simulink model "series"  (R2020a)
settings: Solver=VariableStepAuto  StartTime=0.0  StopTime=5  RelTol=1e-3
settings Model: Creator=ch17d012  LastModifiedBy=ch17d012

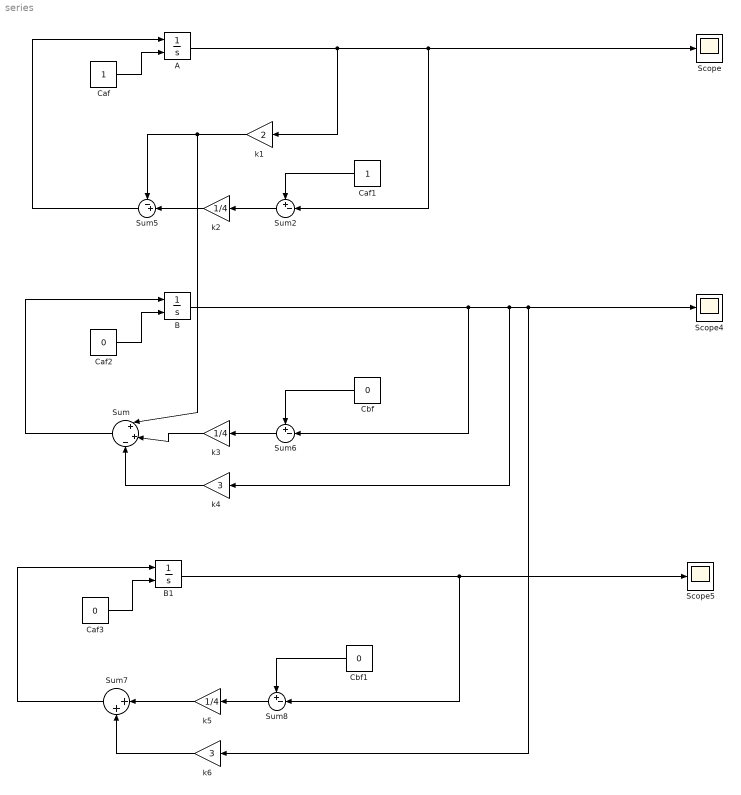
== system series ==
  A : Integrator  InitialConditionSource=external
  B : Integrator  InitialConditionSource=external
  B1 : Integrator  InitialConditionSource=external
  Caf : Constant
  Caf1 : Constant
  Caf2 : Constant  Value=0
  Caf3 : Constant  Value=0
  Cbf : Constant  Value=0
  Cbf1 : Constant  Value=0
  Scope : Scope
  Scope4 : Scope
  Scope5 : Scope
  Sum : Sum  Inputs=|+|+|-
  Sum2 : Sum  Inputs=+-|
  Sum5 : Sum  Inputs=-+|
  Sum6 : Sum  Inputs=+-|
  Sum7 : Sum  Inputs=|++
  Sum8 : Sum  Inputs=+-|
  k1 : Gain  Gain=2
  k2 : Gain  Gain=1/4
  k3 : Gain  Gain=1/4
  k4 : Gain  Gain=3
  k5 : Gain  Gain=1/4
  k6 : Gain  Gain=3
  wires:
  A/1 -> k1/1, Sum2/2, Scope/1
  Caf/1 -> A/2
  Caf1/1 -> Sum2/1
  Sum2/1 -> k2/1
  k1/1 -> Sum/1, Sum5/1
  k2/1 -> Sum5/2
  Sum5/1 -> A/1
  B/1 -> Sum6/2, k4/1, k6/1, Scope4/1
  Cbf/1 -> Sum6/1
  Sum6/1 -> k3/1
  k3/1 -> Sum/2
  k4/1 -> Sum/3
  Sum/1 -> B/1
  Caf2/1 -> B/2
  B1/1 -> Sum8/2, Scope5/1
  Caf3/1 -> B1/2
  Sum7/1 -> B1/1
  Sum8/1 -> k5/1
  Cbf1/1 -> Sum8/1
  k6/1 -> Sum7/2
  k5/1 -> Sum7/1
